simulink subsystem "Thruster_Solver_Mathmatical"  (R2023a)
settings: Solver=VariableStepAuto  StartTime=0.0  StopTime=10.0  RelTol=1e-3

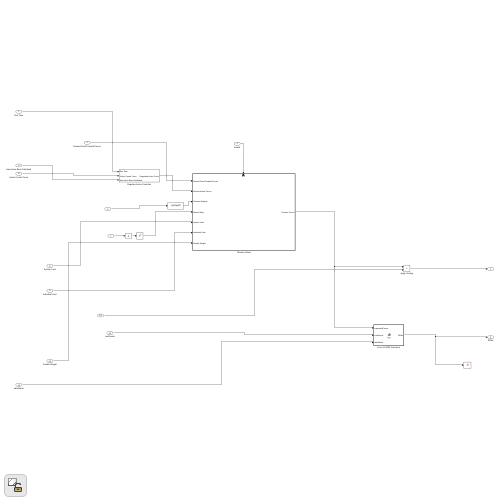
[thumbnail: Simulink's stored preview of the top-level diagram]
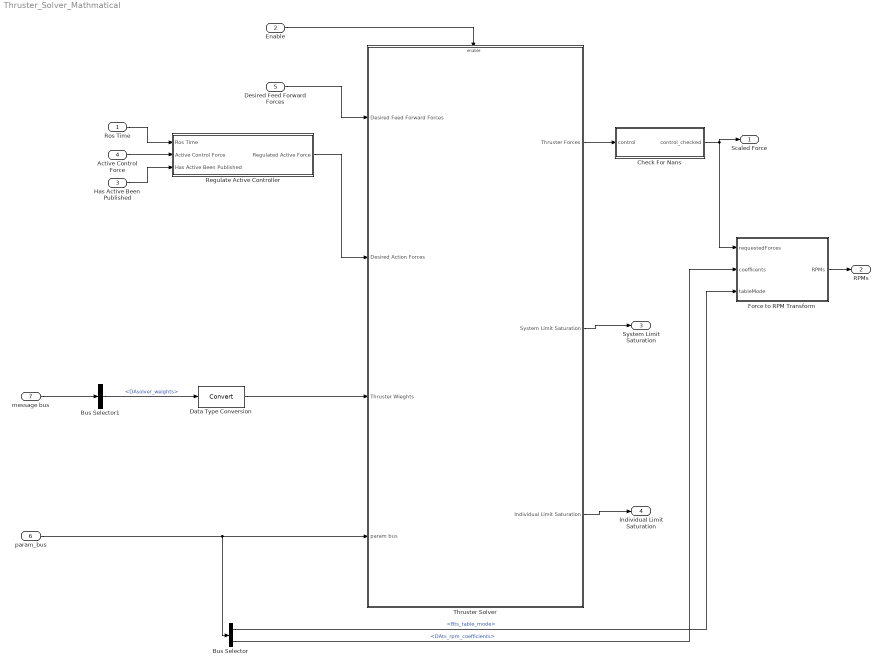
== system Thruster_Solver_Mathmatical ==
  Ros Time : Inport
  Enable : Inport  Port=2
  Has Active Been Published : Inport  Port=3
  Active Control Force : Inport  Port=4
  Desired Feed Forward Forces : Inport  Port=5
  param_bus : Inport  Port=6
  message bus : Inport  Port=7
  Bus Selector : BusSelector  OutputSignals=Bts_table_mode,DAts_rpm_coefficients
  Bus Selector1 : BusSelector  OutputSignals=thruster_solver.DAsolver_weights
  Check For Nans : MATLAB Function  TreatAsAtomicUnit=on
  Data Type Conversion : DataTypeConversion  SaturateOnIntegerOverflow=off  RndMeth=Floor
  Force to RPM Transform : MATLAB Function  TreatAsAtomicUnit=on
  Regulate Active Controller : Subsystem
  Thruster Solver : Subsystem
  Scaled Force : Outport
  RPMs : Outport  Port=2
  System Limit Saturation : Outport  Port=3
  Individual Limit Saturation : Outport  Port=4
  wires:
  Check For Nans/1(control_checked) -> Force to RPM Transform/1(requestedForces), Scaled Force/1
  Thruster Solver/3(Individual Limit Saturation) -> Individual Limit Saturation/1
  Ros Time/1 -> Regulate Active Controller/1(Ros Time)
  Thruster Solver/2(System Limit Saturation) -> System Limit Saturation/1
  Active Control Force/1 -> Regulate Active Controller/2(Active Control Force)
  Has Active Been Published/1 -> Regulate Active Controller/3(Has Active Been Published)
  Force to RPM Transform/1(RPMs) -> RPMs/1
  Regulate Active Controller/1(Regulated Active Force) -> Thruster Solver/2(Desired Action Forces)
  Enable/1 -> Thruster Solver/Enable
  Desired Feed Forward Forces/1 -> Thruster Solver/1(Desired Feed Forward Forces)
  Thruster Solver/1(Thruster Forces) -> Check For Nans/1(control)
  param_bus/1 -> Thruster Solver/4(param bus), Bus Selector/1
  Bus Selector/1 -> Force to RPM Transform/3(tableMode)  "<Bts_table_mode>"
  Bus Selector/2 -> Force to RPM Transform/2(coefficents)  "<DAts_rpm_coefficients>"
  message bus/1 -> Bus Selector1/1
  Bus Selector1/1 -> Data Type Conversion/1  "<DAsolver_weights>"
  Data Type Conversion/1 -> Thruster Solver/3(Thruster Wieghts)

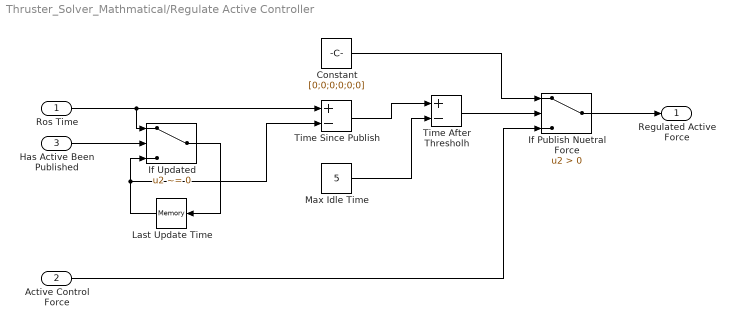
== system Thruster_Solver_Mathmatical/Regulate Active Controller ==
  Ros Time : Inport
  Active Control Force : Inport  Port=2
  Has Active Been Published : Inport  Port=3
  Constant : Constant  Value=[0;0;0;0;0;0]
  If Publish Nuetral Force : Switch  Criteria=u2 > Threshold  SaturateOnIntegerOverflow=off  InputSameDT=off
  If Updated : Switch  Criteria=u2 ~= 0  SaturateOnIntegerOverflow=off  InputSameDT=off
  Last Update Time : Memory
  Max Idle Time : Constant  Value=5
  Time After Thresholh : Sum  Inputs=+-
  Time Since Publish : Sum  Inputs=+-
  Regulated Active Force : Outport
  wires:
  Time After Thresholh/1 -> If Publish Nuetral Force/2
  Max Idle Time/1 -> Time After Thresholh/2
  If Publish Nuetral Force/1 -> Regulated Active Force/1
  Time Since Publish/1 -> Time After Thresholh/1
  Active Control Force/1 -> If Publish Nuetral Force/3
  If Updated/1 -> Last Update Time/1
  Constant/1 -> If Publish Nuetral Force/1
  Has Active Been Published/1 -> If Updated/2
  Last Update Time/1 -> Time Since Publish/2, If Updated/3
  Ros Time/1 -> If Updated/1, Time Since Publish/1

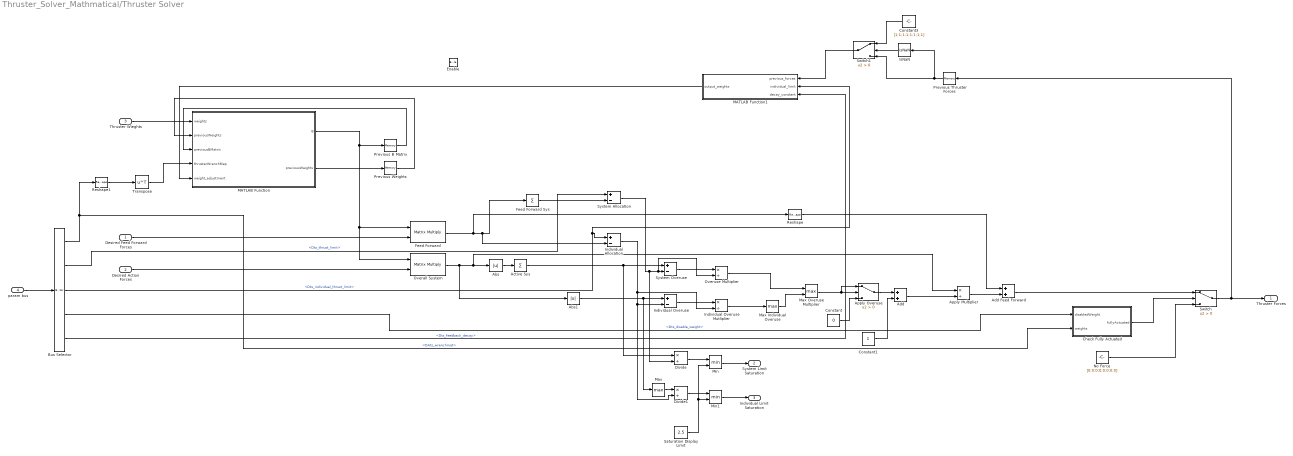
== system Thruster_Solver_Mathmatical/Thruster Solver ==
  Desired Feed Forward Forces : Inport  PortDimensions=[6 1]
  Desired Action Forces : Inport  Port=2  PortDimensions=[6 1]
  Thruster Wieghts : Inport  Port=3  PortDimensions=[8 1]
  param bus : Inport  Port=4
  Enable : EnablePort
  Abs : Abs  SaturateOnIntegerOverflow=off
  Abs1 : Abs  SaturateOnIntegerOverflow=off
  Active Sys : Sum  Inputs=+
  Add : Sum
  Add Feed Forward : Sum  AccumDataTypeStr=double
  Apply Multiplier : Product  Inputs=*/  OutDataTypeStr=double
  Apply Overuse : Switch  Criteria=u2 > Threshold  SaturateOnIntegerOverflow=off  InputSameDT=off
  Bus Selector : BusSelector  OutputSignals=DAts_wrenchmat,Dts_thrust_limit,Dts_individual_thrust_limit,Dts_disable_weight,Dts_feedback_decay
  Check Fully Actuated : MATLAB Function  TreatAsAtomicUnit=on
  Constant : Constant  Value=0
  Constant1 : Constant
  Constant3 : Constant  Value=[1;1;1;1;1;1;1;1]
  Divide : Product  Inputs=*/
  Divide1 : Product  Inputs=*/
  "Feed Forward " : Product  Multiplication=Matrix(*)
  Feed Forward Sys : Sum  Inputs=+
  Individual Allocation : Sum  Inputs=+-
  Individual Overuse : Sum  Inputs=+-
  Individual Overuse Mutliplier : Product  Inputs=*/
  IsNaN : RelationalOperator  Operator=isNaN  OutDataTypeStr=boolean  RndMeth=Simplest  InputSameDT=off
  MATLAB Function : MATLAB Function  TreatAsAtomicUnit=on
  MATLAB Function1 : MATLAB Function  TreatAsAtomicUnit=on
  Max : MinMax  Function=max
  Max Individual Overuse : MinMax  Function=max
  Max Overuse Multiplier : MinMax  Function=max  Inputs=2
  Min : MinMax  Inputs=2
  Min1 : MinMax  Inputs=2
  No Force : Constant  Value=[0;0;0;0;0;0;0;0]
  Overall System : Product  Multiplication=Matrix(*)
  Overuse Multiplier : Product  Inputs=*/
  Previous B Matrix : Memory  InitialCondition=[inf inf inf inf inf inf; inf inf inf inf inf inf; inf inf inf inf inf inf; inf inf inf inf inf inf; inf inf inf inf inf inf; inf inf inf inf inf inf; inf inf inf inf inf inf; inf inf inf inf inf inf]  InheritSampleTime=on
  Previous Thruster Forces : Memory  InitialCondition=[1;1;1;1;1;1;1;1]
  Previous Weights : Memory  InitialCondition=[ inf inf inf inf inf inf inf inf]  InheritSampleTime=on
  Reshape : Reshape  OutputDimensionality=Column vector (2-D)
  Reshape1 : Reshape  OutputDimensionality=Customize  OutputDimensions=[6,8]
  Saturation Display Limit : Constant  Value=2.5
  Switch : Switch  Criteria=u2 > Threshold  SaturateOnIntegerOverflow=off  InputSameDT=off
  Switch1 : Switch  Criteria=u2 > Threshold  SaturateOnIntegerOverflow=off  InputSameDT=off
  System Allocation : Sum  Inputs=+-
  System Overuse : Sum  Inputs=+-
  Transpose : Math  Operator=transpose
  Thruster Forces : Outport
  System Limit Saturation : Outport  Port=2
  Individual Limit Saturation : Outport  Port=3
  wires:
  Transpose/1 -> MATLAB Function/4(thrusterWrenchMap)
  Bus Selector/1 -> Check Fully Actuated/2(weights), Reshape1/1  "<DAts_wrenchmat>"
  Reshape1/1 -> Transpose/1
  param bus/1 -> Bus Selector/1
  Switch1/1 -> MATLAB Function1/1(previous_forces)
  Constant3/1 -> Switch1/1
  IsNaN/1 -> Switch1/2
  Previous Thruster Forces/1 -> IsNaN/1, Switch1/3
  MATLAB Function1/1(output_weights) -> MATLAB Function/5(weight_adjustment)
  MATLAB Function/2(previousWeights) -> Previous Weights/1
  Previous Weights/1 -> MATLAB Function/2("previousWeights ")
  Bus Selector/5 -> MATLAB Function1/3(decay_constant)  "<Dts_feedback_decay>"
  Active Sys/1 -> System Overuse/1, Divide/1
  Abs/1 -> Active Sys/1
  Abs1/1 -> Individual Overuse/1, Max/1
  Max/1 -> Divide1/1
  Min1/1 -> Individual Limit Saturation/1
  Divide1/1 -> Min1/1
  Min/1 -> System Limit Saturation/1
  Saturation Display Limit/1 -> Min/2, Min1/2
  Divide/1 -> Min/1
  Constant/1 -> Apply Overuse/3
  Feed Forward Sys/1 -> System Allocation/2
  Individual Overuse/1 -> Individual Overuse Mutliplier/1
  Individual Allocation/1 -> Individual Overuse Mutliplier/2, Individual Overuse/2, Divide1/2
  Overall System/1 -> Abs1/1, Apply Multiplier/1, Abs/1
  Max Overuse Multiplier/1 -> Apply Overuse/1, Apply Overuse/2
  Desired Feed Forward Forces/1 -> "Feed Forward "/2
  System Overuse/1 -> Overuse Multiplier/1
  Apply Multiplier/1 -> Add Feed Forward/2
  Overuse Multiplier/1 -> Max Overuse Multiplier/1
  Max Individual Overuse/1 -> Max Overuse Multiplier/2
  System Allocation/1 -> Overuse Multiplier/2, System Overuse/2, Divide/2
  Desired Action Forces/1 -> Overall System/2
  "Feed Forward "/1 -> Reshape/1, Individual Allocation/2, Feed Forward Sys/1
  Constant1/1 -> Add/2
  Individual Overuse Mutliplier/1 -> Max Individual Overuse/1
  Apply Overuse/1 -> Add/1
  Add/1 -> Apply Multiplier/2
  Add Feed Forward/1 -> Switch/1
  MATLAB Function/1(B) -> Overall System/1, "Feed Forward "/1, Previous B Matrix/1
  Previous B Matrix/1 -> MATLAB Function/3(previousBMatrix)
  Thruster Wieghts/1 -> MATLAB Function/1(weights)
  Bus Selector/2 -> System Allocation/1  "<Dts_thrust_limit>"
  Bus Selector/3 -> Individual Allocation/1, MATLAB Function1/2(individual_limit)  "<Dts_individual_thrust_limit>"
  Reshape/1 -> Add Feed Forward/1
  Check Fully Actuated/1(fullyActuated) -> Switch/2
  Bus Selector/4 -> Check Fully Actuated/1(disabledWeight)  "<Dts_disable_weight>"
  No Force/1 -> Switch/3
  Switch/1 -> Thruster Forces/1, Previous Thruster Forces/1

== matlab function Thruster_Solver_Mathmatical/Force to RPM Transform ==
function RPMs = fcn(requestedForces, coefficents, tableMode)

%the output array with rpm values
RPMs = zeros([8,1]);

if(tableMode)
   %evaluate each thruster -- discontinuos curve
    for i = 1:8
        requestedForce = requestedForces(i);
        RPMs(i) = ((-500 * exp((-1/2) * abs(requestedForce))) + 500) * sign(requestedForce);
    end 

else

    %evaluate each thruster -- discontinuos curve
    for i = 1:8
        requestedForce = requestedForces(i);
        
        if(requestedForce > 0)
            %positive curve
            RPMs(i) = round(coefficents(1) + coefficents(2) * requestedForces(i) + coefficents(3) * tanh(requestedForces(i)) + requestedForces(i)^(1/4) * coefficents(4));
        else
            %negative curve
            RPMs(i) = round(coefficents(5) + coefficents(6) * requestedForces(i) + coefficents(7) * tanh(requestedForces(i)) + abs(requestedForces(i))^(1/4) * coefficents(8));
        end
    
    end

end

== matlab function Thruster_Solver_Mathmatical/Thruster Solver/Check Fully Actuated ==
function fullyActuated = fcn(disabledWeight, weights)

enabled_thrusters = 0;

%count number of enabled thrusters
for i = 1:length(weights)
    if(weights(i) < disabledWeight)
        enabled_thrusters = enabled_thrusters + 1;
    end
end

%if enough thrusters to be fully actuated allow forces
if(enabled_thrusters >= 6)
    fullyActuated = 1;

    return
end

fullyActuated = 0;

== matlab function Thruster_Solver_Mathmatical/Thruster Solver/MATLAB Function ==
function [B,previousWeights] = generateBMatrix(weights, previousWeights, previousBMatrix, thrusterWrenchMap, weight_adjustment)

    adjusted_weights = weights .* weight_adjustment;

    if(isequal(weights, previousWeights) && ~isnan(previousBMatrix(1,1)))
        %if the weights are the same, just send the previous B matrix
        B = previousBMatrix;
        previousWeights = weights;
        return
    end


    %if new weights, calculate the a new b matrix
    weightsMatrix = diag(adjusted_weights);
    B = inv(weightsMatrix) * (thrusterWrenchMap) * inv((transpose(thrusterWrenchMap) * inv(weightsMatrix) * (thrusterWrenchMap)));
    previousWeights = weights;
    
end

== matlab function Thruster_Solver_Mathmatical/Check For Nans ==
function control_checked = stopNans(control)

control_checked = zeros(8,1);

%loop through and asign non nans
for i=1:8
    if(~isnan(control(i)))
        control_checked(i) = control(i);
    end
end

== matlab function Thruster_Solver_Mathmatical/Thruster Solver/MATLAB Function1 ==
function output_weights = fcn(previous_forces, individual_limit, decay_constant)

output_weights = (previous_forces ./ individual_limit + 1) .^ (-1*decay_constant);
